simulink model "adapptiveController"  (R2024a)
settings: Solver=ode1  StartTime=0.0  StopTime=10  FixedStep=0.01  RelTol=1e-3
libraries: robotmaniplib x1
settings Model: Creator=gujun  LastModifiedBy=gujun
settings RTWCC: GPUComputeCapability=3.5

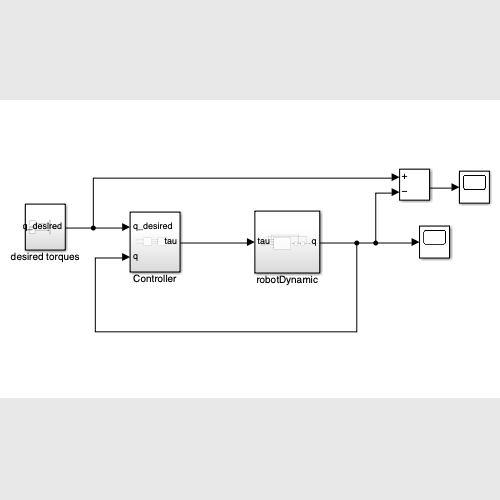
[thumbnail: Simulink's stored preview of the top-level diagram]
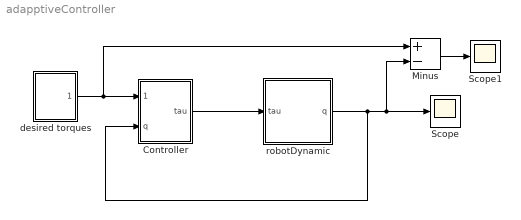
== system adapptiveController ==
  Controller : Subsystem
  Minus : Sum  Inputs=+-
  Scope : Scope
  Scope1 : Scope
  desired torques : Subsystem
  robotDynamic : Subsystem
  wires:
  robotDynamic/1(q) -> Minus/2, Scope/1, Controller/2(q)
  desired torques/1(q_desired) -> Minus/1, Controller/1(q_desired)
  Controller/1(tau) -> robotDynamic/1(tau)
  Minus/1 -> Scope1/1

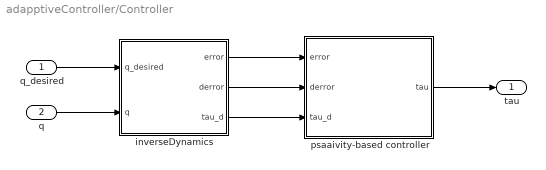
== system adapptiveController/Controller ==
  q_desired : Inport
  q : Inport  Port=2
  inverseDynamics : Subsystem
  psaaivity-based controller : MATLAB Function  TreatAsAtomicUnit=on
  tau : Outport
  wires:
  q_desired/1 -> inverseDynamics/1(q_desired)
  inverseDynamics/3(tau_d) -> psaaivity-based controller/3(tau_d)
  psaaivity-based controller/1(tau) -> tau/1
  q/1 -> inverseDynamics/2(q)
  inverseDynamics/1(error) -> psaaivity-based controller/1(error)
  inverseDynamics/2(derror) -> psaaivity-based controller/2(derror)

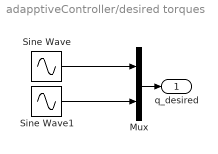
== system adapptiveController/desired torques ==
  Mux : Mux  Inputs=2
  Sine Wave : Sin  SampleTime=0
  Sine Wave1 : Sin  Bias=pi/2  SampleTime=0
  q_desired : Outport
  wires:
  Mux/1 -> q_desired/1
  Sine Wave1/1 -> Mux/2
  Sine Wave/1 -> Mux/1

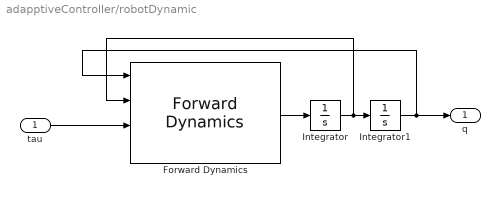
== system adapptiveController/robotDynamic ==
  tau : Inport
  Forward Dynamics : robotmaniplib/Forward Dynamics  RigidBodyTree=twoJointRigidBodyTree  SimulateUsing=Interpreted execution
  Integrator : Integrator
  Integrator1 : Integrator
  q : Outport
  wires:
  Forward Dynamics/1 -> Integrator/1
  tau/1 -> Forward Dynamics/3
  Integrator1/1 -> Forward Dynamics/1, q/1
  Integrator/1 -> Forward Dynamics/2, Integrator1/1

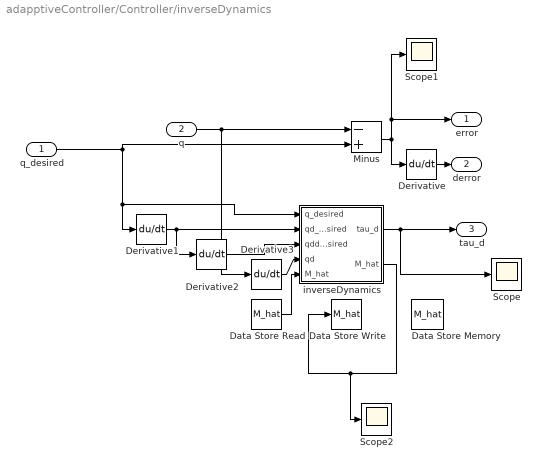
== system adapptiveController/Controller/inverseDynamics ==
  q_desired : Inport
  q : Inport  Port=2
  Data Store Memory : DataStoreMemory  DataStoreName=M_hat  WriteAfterWriteMsg=warning  InitialValue=[1, 0; 0,1;]  ShowAdditionalParam=off
  Data Store Read : DataStoreRead  DataStoreName=M_hat  IndexOptions=Index vector (dialog)  Indices=1  OutputSizes=1
  Data Store Write : DataStoreWrite  DataStoreName=M_hat  IndexOptions=Index vector (dialog)  Indices=1  OutputSizes=1
  Derivative{,1..3} (4 alike) : Derivative
  Minus : Sum  Inputs=-+
  Scope : Scope
  Scope1 : Scope
  Scope2 : Scope
  inverseDynamics : MATLAB Function  TreatAsAtomicUnit=on
  error : Outport
  derror : Outport  Port=2
  tau_d : Outport  Port=3
  wires:
  inverseDynamics/1(tau_d) -> Scope/1, tau_d/1
  Derivative/1 -> derror/1
  Derivative1/1 -> Derivative2/1, inverseDynamics/2(qd_desired)
  q_desired/1 -> Minus/2, inverseDynamics/1(q_desired), Derivative1/1
  Derivative2/1 -> inverseDynamics/3(qdd_desired)
  Minus/1 -> error/1, Scope1/1, Derivative/1
  Derivative3/1 -> inverseDynamics/4(qd)
  q/1 -> Derivative3/1, Minus/1
  Data Store Read/1 -> inverseDynamics/5("M_hat ")
  inverseDynamics/2(M_hat) -> Scope2/1, Data Store Write/1

== matlab function adapptiveController/Controller/psaaivity-based controller ==
  data: error input; tau output; derror input; tau_d input
function tau = controller(error, derror, tau_d)

kp = [300, 0;
       0, 300];


kd = [50, 0;
        0, 50];

tau = kp * error + kd * derror + tau_d;

== matlab function adapptiveController/Controller/inverseDynamics/inverseDynamics ==
  data: tau_d output; q_desired input; qd_desired input; qdd_desired input; qd input; M_hat input; M_hat output
function [tau_d, M_hat]  = dynamics(q_desired, qd_desired, qdd_desired, qd, M_hat)


I1 = 0.05;
m1 = 1.5;
lg1 = 0.2;
lr1 = lg1 / 2;

I2 = 0.01;
m2 = 0.5;
lg2 = 0.2;
lr2 = lg2 / 2;

gamma = 0.1;

g = 9.8;

M_hat = M_hat + gamma * (qdd_desired .* (qd_desired - qd));

V = [-m2 * lg1 * lr2 * qd_desired(2)^2 * sin(q_desired(2));
    m2 * lg1 * lr2 * qd_desired(1)^2 * sin(q_desired(2))];

G = [m1 * g * lr1 * cos(q_desired(1)) + m2 * g * lg1 * cos(q_desired(1));
    m2 * g * lr2 * cos(q_desired(1) + q_desired(2));];

tau_d = M_hat * qdd_desired + V + G;

end
